simulink model "hdlcoder_streaming_mat_inv_max_lat_cholesky"  (R2021a)
settings: Solver=FixedStepDiscrete  StartTime=0.0  StopTime=1000  RelTol=1e-3
InitFcn:
  | arow = 6;
  | acol  = 6;
libraries: hdlsllib x2, simulink x1
settings Model: DataTypeOverride=Off  PauseTimes=60  Creator=The MathWorks, Inc.  LastModifiedBy=ffn
settings SolverCC: AlgebraicLoopSolver=TrustRegion
settings DataIOCC: SaveOutput=off  SaveTime=off  ReturnWorkspaceOutputs=off
settings OptimizationCC: BlockReduction=off  ConditionallyExecuteInputs=off  DefaultParameterBehavior=Inlined
settings DebuggingCC: AlgebraicLoopMsg=error  SingleTaskRateTransMsg=error  IntegerOverflowMsg=none  ParameterPrecisionLossMsg=none  PregeneratedLibrarySubsystemCodeDiagnostic=none  SFMachineParentedDataDiag=warning  ArithmeticOperatorsInVariantConditions=warning
settings HardwareCC: ProdBitPerPointer=32  ProdBitPerSizeT=32  ProdBitPerPtrDiffT=32  ProdLargestAtomicFloat=None  ProdIntDivRoundTo=Undefined  ProdEndianess=Unspecified  ProdWordSize=32  ProdHWDeviceType=ASIC/FPGA->ASIC/FPGA  ProdEqTarget=off
settings SFSimCC: SimUseLocalCustomCode=off
settings RTWCC: RTWUseLocalCustomCode=off
settings CodeAppCC: StateflowObjectComments=on

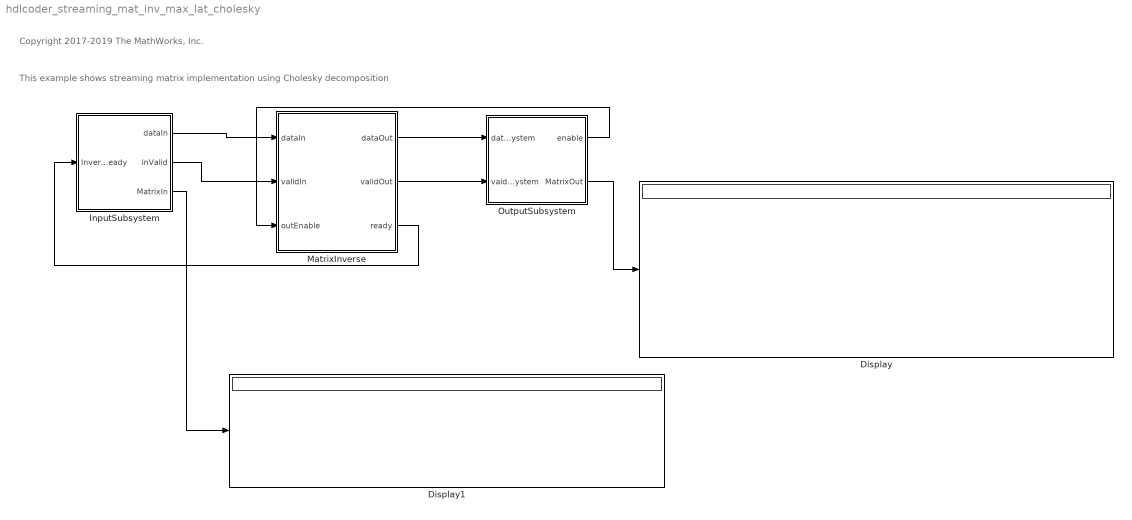
== system hdlcoder_streaming_mat_inv_max_lat_cholesky ==
  note: This example shows streaming matrix implementation using Cholesky decomposition
  note: Copyright 2017-2019 The MathWorks, Inc.
  Display : Display
  Display1 : Display
  InputSubsystem : Subsystem  Description=|
      | This block will generate serialized aValid and aData signals using transpose math function,
      | Reshape block,Serializer. These aValid,aData are the inputs for MatInverse subsystem.
  MatrixInverse : Subsystem
  OutputSubsystem : Subsystem  Description=|
      | This block contains Deserializer,Reshape block, transpose math function to create a 4x4 matrix from
      | cData when cValid is enabled and also contains comparision logic betweem Matlab System block of 
      | MatrixInverse and HDL compatible implementation block of MatrixInverse.
  wires:
  InputSubsystem/1(dataIn) -> MatrixInverse/1(dataIn)
  OutputSubsystem/1(enable) -> MatrixInverse/3(outEnable)
  InputSubsystem/2(inValid) -> MatrixInverse/2(validIn)
  MatrixInverse/1(dataOut) -> OutputSubsystem/1(dataSystem)
  MatrixInverse/3(ready) -> InputSubsystem/1(InverseReady)
  MatrixInverse/2(validOut) -> OutputSubsystem/2(vaidInSystem)
  OutputSubsystem/2(MatrixOut) -> Display/1
  InputSubsystem/3(MatrixIn) -> Display1/1

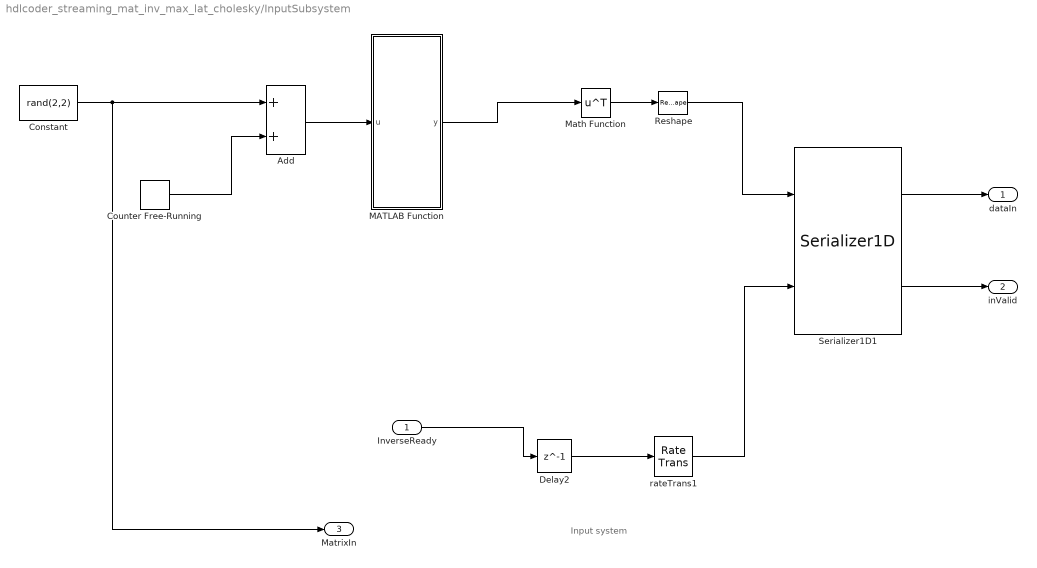
== system hdlcoder_streaming_mat_inv_max_lat_cholesky/InputSubsystem ==
  note: Input system
  InverseReady : Inport
  Add : Sum  OutDataTypeStr=single
  Constant : Constant  Value=rand(2,2)
  Counter Free-Running : simulink/Sources/Counter Free-Running  NumBits=16  tsamp=1
  Delay2 : Delay  DelayLength=1
  MATLAB Function : MATLAB Function  TreatAsAtomicUnit=on
  Math Function : Math  Operator=transpose  SignedPower=on  SaturateOnIntegerOverflow=on
  Reshape : Reshape
  Serializer1D1 : hdlsllib/HDL Operations/Serializer1D  Ratio=arow*acol  IdleCycles=0  validIn=on  startOut=off  validOut=on  inputDataDimensions=-1  inputSampleTime=-1  inputSignalType=auto
      settings: SourceProductBaseCode=SL
  rateTrans1 : RateTransition  Integrity=off  OutPortSampleTimeOpt=Multiple of input port sample time  OutPortSampleTimeMultiple=arow*acol  OutPortSampleTime=1
  dataIn : Outport  VectorParamsAs1DForOutWhenUnconnected=off
  inValid : Outport  Port=2  VectorParamsAs1DForOutWhenUnconnected=off
  MatrixIn : Outport  Port=3
  wires:
  Math Function/1 -> Reshape/1
  Serializer1D1/1 -> dataIn/1
  rateTrans1/1 -> Serializer1D1/2
  Serializer1D1/2 -> inValid/1
  Reshape/1 -> Serializer1D1/1
  Delay2/1 -> rateTrans1/1
  MATLAB Function/1(y) -> Math Function/1
  Constant/1 -> MatrixIn/1, Add/1
  Counter Free-Running/1 -> Add/2
  Add/1 -> MATLAB Function/1(u)
  InverseReady/1 -> Delay2/1

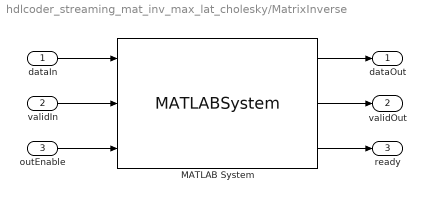
== system hdlcoder_streaming_mat_inv_max_lat_cholesky/MatrixInverse ==
  dataIn : Inport
  validIn : Inport  Port=2
  outEnable : Inport  Port=3
  MATLAB System : MATLABSystem  System=hdl.MatrixInverse  MatrixSize=2  LatencyStrategyType=MAX  AlgorithmType=GaussJordanElimination  SimulateUsing=Code generation
      mask Type: hdl.MatrixInverse
      mask Display:
      | disp(['MatrixInverse:Gauss-Jordan' char(10) ' processingLatency: 208']);
      | port_label('input',1,'dataIn');
      | port_label('input',2,'validIn');
      | port_label('input',3,'outEnable');
      | port_label('output',1,'dataOut');
      | port_label('output',2,'validOut');
      | port_label('output',3,'ready');
  dataOut : Outport  VectorParamsAs1DForOutWhenUnconnected=off
  validOut : Outport  Port=2  VectorParamsAs1DForOutWhenUnconnected=off
  ready : Outport  Port=3  VectorParamsAs1DForOutWhenUnconnected=off
  wires:
  MATLAB System/2 -> validOut/1
  dataIn/1 -> MATLAB System/1
  MATLAB System/3 -> ready/1
  MATLAB System/1 -> dataOut/1
  outEnable/1 -> MATLAB System/3
  validIn/1 -> MATLAB System/2

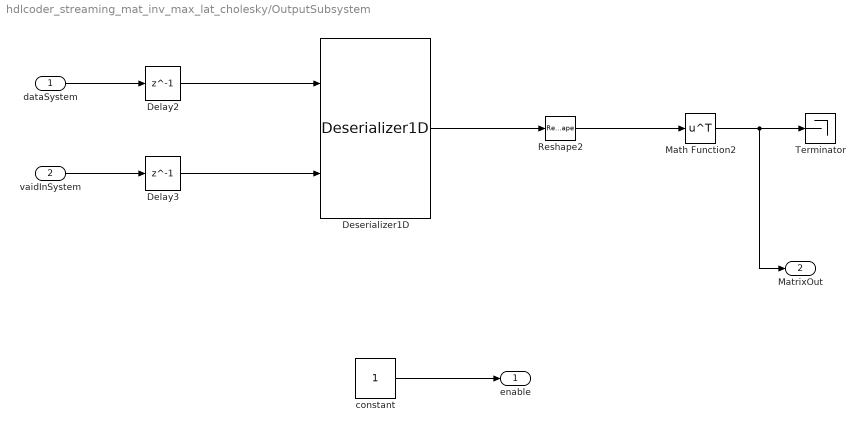
== system hdlcoder_streaming_mat_inv_max_lat_cholesky/OutputSubsystem ==
  dataSystem : Inport
  vaidInSystem : Inport  Port=2
  Delay2 : Delay  DelayLength=1
  Delay3 : Delay  DelayLength=1
  Deserializer1D : hdlsllib/HDL Operations/Deserializer1D  Ratio=arow*acol  IdleCycles=0  InitialCondition=0  startIn=off  validIn=on  validOut=off  inputDataDimensions=-1  inputSampleTime=-1  inputSignalType=auto
      settings: SourceProductBaseCode=SL
  Math Function2 : Math  Operator=transpose  SignedPower=on  SaturateOnIntegerOverflow=on
  Reshape2 : Reshape  OutputDimensionality=Customize  OutputDimensions=[arow acol]
  Terminator : Terminator
  constant : Constant  OutDataTypeStr=boolean  SampleTime=-1
  enable : Outport  VectorParamsAs1DForOutWhenUnconnected=off
  MatrixOut : Outport  Port=2  VectorParamsAs1DForOutWhenUnconnected=off
  wires:
  constant/1 -> enable/1
  Reshape2/1 -> Math Function2/1
  Delay3/1 -> Deserializer1D/2
  dataSystem/1 -> Delay2/1
  vaidInSystem/1 -> Delay3/1
  Math Function2/1 -> MatrixOut/1, Terminator/1
  Delay2/1 -> Deserializer1D/1
  Deserializer1D/1 -> Reshape2/1

== matlab function hdlcoder_streaming_mat_inv_max_lat_cholesky/InputSubsystem/MATLAB Function ==
  data: u input; y output
function y = fcn(u)

[arow, acol] = size(u);
defPosDefMat = single(ones(arow,acol));
for i = 1:arow
   for j = 1:acol
       if(i ==j)
           defPosDefMat(i,j) = i;
       end
   end    
end    
A = u; 
A = 0.5*(A+A');
A = A*A';
resPosDefMat = A + arow*eye(arow);
eigVal = eig(resPosDefMat);
if issymmetric(resPosDefMat) && isempty(eigVal(eigVal<=0))
 y = resPosDefMat;
else
 y = defPosDefMat;    
end
